simulink model "SignalProcessing3"  (R2019b)
settings: Solver=VariableStepAuto  StartTime=0.0  StopTime=5  RelTol=1e-3
libraries: dspsigops x4, dspstat3 x4, simulink x2, dspfdesign x1
settings Model: Creator=Ege  LastModifiedBy=90534
settings DataIOCC: ReturnWorkspaceOutputs=off
settings DebuggingCC: ArithmeticOperatorsInVariantConditions=warning
settings SFSimCC: SimUseLocalCustomCode=off  CustomCodeUndefinedFunction=UseInterfaceOnly
settings RTWCC: RTWUseLocalCustomCode=off
settings CodeAppCC: StateflowObjectComments=on

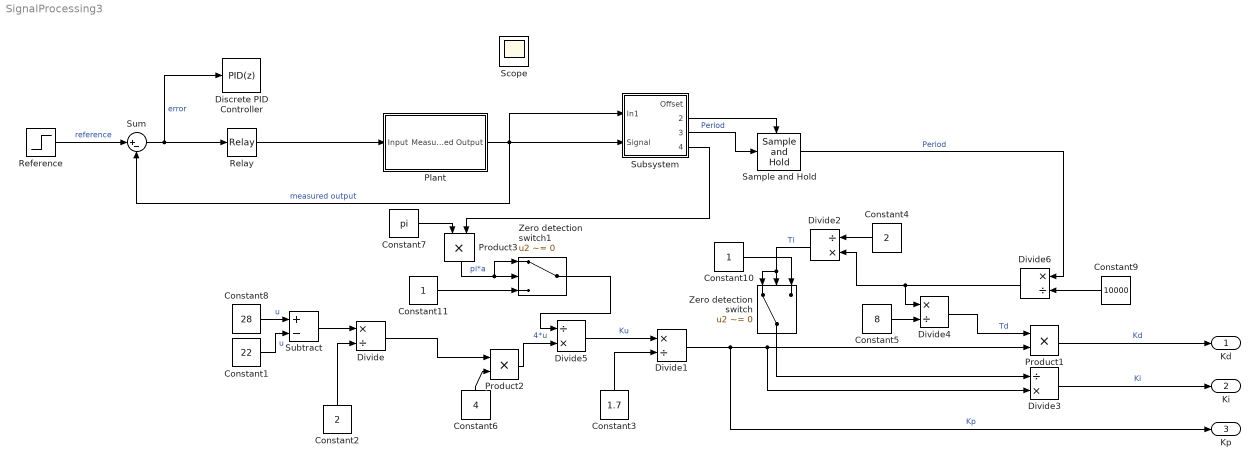
== system SignalProcessing3 ==
  Constant1 : Constant  Value=22
  Constant10 : Constant
  Constant11 : Constant
  Constant2 : Constant  Value=2
  Constant3 : Constant  Value=1.7
  Constant4 : Constant  Value=2
  Constant5 : Constant  Value=8
  Constant6 : Constant  Value=4
  Constant7 : Constant  Value=pi
  Constant8 : Constant  Value=28
  Constant9 : Constant  Value=10000
  Discrete PID Controller : simulink/Continuous/PID Controller  Controller=PID  Form=Parallel  TimeDomain=Discrete-time  SampleTime=-1  IntegratorMethod=Forward Euler  FilterMethod=Forward Euler  ControllerParametersSource=internal  P=27.5252785714347  I=242.974803591307  D=0.637793516322299  UseFilter=off  N=9773.41340021372  TunerSelectOption=Transfer Function Based (PID Tuner App)  InitialConditionSource=internal  InitialConditionForIntegrator=0  InitialConditionForFilter=0  DifferentiatorICPrevScaledInput=0  ExternalReset=none  TrackingMode=off  Kt=1  LimitOutput=off  UpperSaturationLimit=inf  LowerSaturationLimit=-inf  LinearizeAsGain=off  AntiWindupMode=none  Kb=1  POutMin=[]  POutMax=[]  IOutMin=[]  IOutMax=[]  DOutMin=[]  DOutMax=[]  NOutMin=[]  NOutMax=[]  SumOutMin=[]  SumOutMax=[]  SaturationOutMin=[]  SaturationOutMax=[]  PParamMin=[]  PParamMax=[]  IParamMin=[]  IParamMax=[]  DParamMin=[]  DParamMax=[]  NParamMin=[]  NParamMax=[]  KbParamMin=[]  KbParamMax=[]  KtParamMin=[]  KtParamMax=[]  KbOutMin=[]  KbOutMax=[]  KtOutMin=[]  KtOutMax=[]  IntegratorOutMin=[]  IntegratorOutMax=[]  FilterOutMin=[]  FilterOutMax=[]  SumI1OutMin=[]  SumI1OutMax=[]  SumI2OutMin=[]  SumI2OutMax=[]  SumI3OutMin=[]  SumI3OutMax=[]  SumI4OutMin=[]  SumI4OutMax=[]  SumDOutMin=[]  SumDOutMax=[]  DifferentiatorOutMin=[]  DifferentiatorOutMax=[]  FilterDiffOutCoefMin=[]  FilterDiffOutCoefMax=[]  ReciprocalOutMin=[]  ReciprocalOutMax=[]  SumDenOutMin=[]  SumDenOutMax=[]  SumNumOutMin=[]  SumNumOutMax=[]  DivideOutMin=[]  DivideOutMax=[]  IntegratorContinuousStateAttributes=''  IntegratorStateMustResolveToSignalObject=off  IntegratorRTWStateStorageClass=Auto  FilterContinuousStateAttributes=''  FilterStateMustResolveToSignalObject=off  FilterRTWStateStorageClass=Auto  ParallelPVariant=InternalParameters  IdealPVariant=Disabled  IVariant=InternalParameters  DVariant=InternalParameters  IntegratorVariant=Discrete  SatVariant=Disabled  AWVariant=Passthrough  PCopyVariant=Disabled  TRVariant=Disabled  FdbkBlocksVariant=Forward  IdealPFdbkVariant=Disabled  SatFdbkVariant=Disabled  DerivativeFilterVariant=Differentiator  NVariant=Passthrough  NCopyVariant=Disabled_SignalSpec  FilterICVariant=InternalICsDifferentiator  IntegratorICVariant=InternalICs  ExternalResetVariant=Disabled  TRSumVariant=Passthrough  SumFdbkVariant=Disabled  SumVariant=Sum_PID
  Divide : Product  Inputs=*/
  Divide1 : Product  Inputs=*/  SaturateOnIntegerOverflow=on  RndMeth=Zero
  Divide2 : Product  Inputs=/*  SaturateOnIntegerOverflow=on  RndMeth=Zero
  Divide3 : Product  Inputs=/*  SaturateOnIntegerOverflow=on  RndMeth=Zero
  Divide4 : Product  Inputs=*/  SaturateOnIntegerOverflow=on  RndMeth=Zero
  Divide5 : Product  Inputs=/*  SaturateOnIntegerOverflow=on  RndMeth=Zero
  Divide6 : Product  Inputs=*/
  Plant : Subsystem
  Product1 : Product
  Product2 : Product
  Product3 : Product
  Reference : Step  After=25  SampleTime=0
  Relay : Relay  OnOutputValue=on  OffOutputValue=off
  Sample and Hold : dspsigops/Sample and Hold  trig=Rising edge  initCond=0  latchinput=off
  Subsystem : Subsystem
  Subtract : Sum  Inputs=+-
  Sum : Sum  Inputs=|+-
  Zero detection switch : Switch  Criteria=u2 ~= 0
  Zero detection switch1 : Switch  Criteria=u2 ~= 0
  Kd : Outport
  "Ki " : Outport  Port=2
  Kp : Outport  Port=3
  Scope : Scope
  wires:
  Subtract/1 -> Divide/1
  Constant1/1 -> Subtract/2  "u"
  Constant8/1 -> Subtract/1  "u"
  Constant2/1 -> Divide/2
  Relay/1 -> Plant/1(Input)
  Sum/1 -> Relay/1, Discrete PID Controller/1  "error"
  Plant/1(Measured Output) -> Subsystem/2("Signal "), Subsystem/1(In1), Sum/2  "measured output"
  Reference/1 -> Sum/1  "reference"
  Constant9/1 -> Divide6/2
  Divide6/1 -> Divide2/2, Divide4/1
  Subsystem/3("Period ") -> Sample and Hold/1  "Period"
  Divide4/1 -> Product1/1  "Td"
  Constant7/1 -> Product3/1
  Product2/1 -> Divide5/2  "4*u"
  Divide2/1 -> Zero detection switch/1, Zero detection switch/2  "Ti"
  Constant4/1 -> Divide2/1
  Constant5/1 -> Divide4/2
  Divide5/1 -> Divide1/1  "Ku"
  Product1/1 -> Kd/1  "Kd"
  Divide1/1 -> Kp/1, Divide3/2, Product1/2  "Kp"
  Product3/1 -> Zero detection switch1/1, Zero detection switch1/2  "pi*a"
  Constant6/1 -> Product2/2
  Divide/1 -> Product2/1
  Constant3/1 -> Divide1/2
  Divide3/1 -> "Ki "/1  "Ki"
  Subsystem/2(Stable) -> Sample and Hold/Trigger
  Sample and Hold/1 -> Divide6/1  "Period"
  Subsystem/4(Amplitude) -> Product3/2
  Constant10/1 -> Zero detection switch/3
  Zero detection switch/1 -> Divide3/1
  Constant11/1 -> Zero detection switch1/3
  Zero detection switch1/1 -> Divide5/1

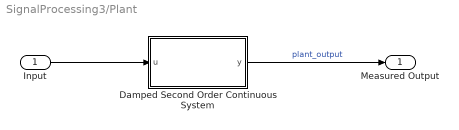
== system SignalProcessing3/Plant ==
  Input : Inport
  Damped Second Order Continuous System : Subsystem  mask{wn=90, zeta=5}
      mask prompts: wn "Undamped natural frequency (wn, rad/s)"; zeta "Damping factor (zeta)"
  Measured Output : Outport
  wires:
  Input/1 -> Damped Second Order Continuous System/1(u)
  Damped Second Order Continuous System/1(y) -> Measured Output/1  "plant_output"

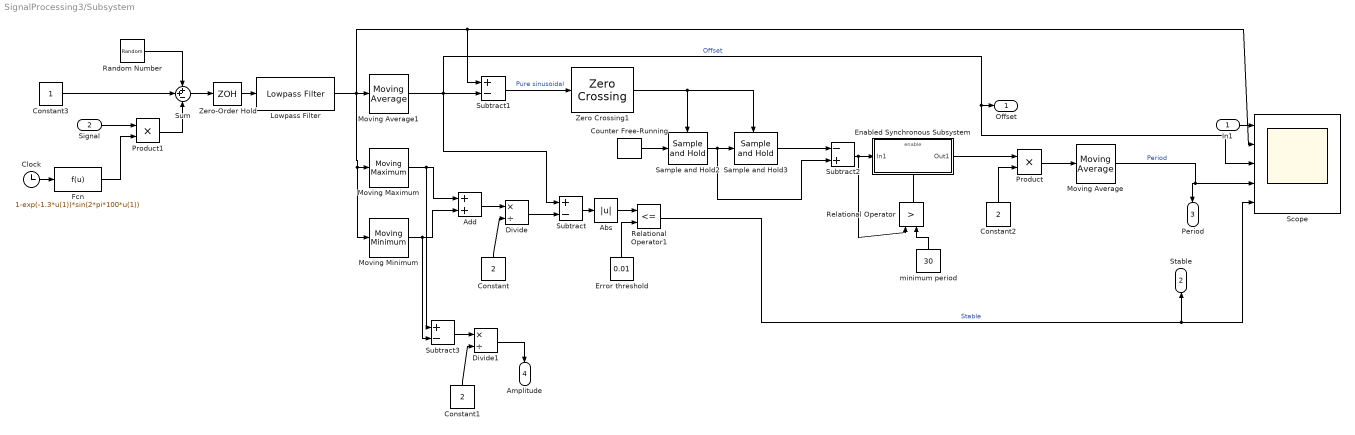
== system SignalProcessing3/Subsystem ==
  In1 : Inport
  "Signal " : Inport  Port=2
  Abs : Abs
  Add : Sum
  Clock : Clock
  Constant : Constant  Value=2
  Constant1 : Constant  Value=2
  Constant2 : Constant  Value=2
  Constant3 : Constant
  Counter Free-Running : simulink/Sources/Counter Free-Running  NumBits=16  tsamp=-1
  Divide : Product  Inputs=*/
  Divide1 : Product  Inputs=*/
  Enabled Synchronous Subsystem : Subsystem  TreatAsAtomicUnit=on
  Error threshold : Constant  Value=0.01
  Fcn : Fcn  Expr=1-exp(-1.3*u(1))*sin(2*pi*100*u(1))
  Lowpass Filter : dspfdesign/Lowpass Filter  FilterType=FIR  DesignForMinimumOrder=on  FilterOrder=50  PassbandFrequency=1e3  StopbandFrequency=2e3  PassbandRipple=0.1  StopbandAttenuation=80  InheritSampleRate=on  SampleRate=44100  SimulateUsing=Interpreted execution  roundingMode=Floor  coeffsDataTypeStr=fixdt(1,16)
  Moving Average : dspstat3/Moving Average  Method=Sliding window  ForgettingFactorPort=off  SpecifyWindowLength=on  WindowLength=10000  ForgettingFactor=0.1  SimulateUsing=Code generation
  Moving Average1 : dspstat3/Moving Average  Method=Sliding window  ForgettingFactorPort=off  SpecifyWindowLength=on  WindowLength=10000  ForgettingFactor=0.1  SimulateUsing=Code generation
  Moving Maximum : dspstat3/Moving Maximum  SpecifyWindowLength=on  WindowLength=10000  SimulateUsing=Code generation
      settings: SourceProductName=DSP System Toolbox  SourceProductBaseCode=DS
  Moving Minimum : dspstat3/Moving Minimum  SpecifyWindowLength=on  WindowLength=10000  SimulateUsing=Code generation
      settings: SourceProductName=DSP System Toolbox  SourceProductBaseCode=DS
  Product : Product
  Product1 : Product
  Random Number : RandomNumber  Variance=0.01  SampleTime=0.0001
  Relational Operator : RelationalOperator  Operator=>  OutDataTypeStr=boolean  RndMeth=Nearest
  Relational Operator1 : RelationalOperator  Operator=<=  OutDataTypeStr=boolean  RndMeth=Simplest
  Sample and Hold2 : dspsigops/Sample and Hold  trig=Rising edge  initCond=0  latchinput=on
  Sample and Hold3 : dspsigops/Sample and Hold  trig=Rising edge  initCond=0  latchinput=on
  Scope : Scope  NumInputPorts=5
  Subtract : Sum  Inputs=+-
  Subtract1 : Sum  Inputs=+-
  Subtract2 : Sum  Inputs=-+  AccumDataTypeStr=fixdt(0,16,0)
  Subtract3 : Sum  Inputs=+-
  Sum : Sum  Inputs=++-
  Zero Crossing1 : dspsigops/Zero Crossing  InputProcessing=Columns as channels (frame based)
      settings: SourceProductName=DSP System Toolbox  SourceProductBaseCode=DS
  Zero-Order Hold : ZeroOrderHold  SampleTime=0.0001
  minimum period : Constant  Value=30
  Offset : Outport
  Stable : Outport  Port=2
  "Period " : Outport  Port=3
  Amplitude : Outport  Port=4
  wires:
  Moving Maximum/1 -> Subtract3/1, Add/1
  Lowpass Filter/1 -> Moving Minimum/1, Moving Maximum/1, Moving Average1/1, Scope/2, Subtract1/1
  Moving Average1/1 -> Offset/1, Scope/3, Subtract/1, Subtract1/2  "Offset"
  Counter Free-Running/1 -> Sample and Hold2/1
  Clock/1 -> Fcn/1
  Sample and Hold2/1 -> Subtract2/2, Sample and Hold3/1
  Divide/1 -> Subtract/2
  Relational Operator1/1 -> Stable/1, Scope/5  "Stable"
  Sample and Hold3/1 -> Subtract2/1
  Subtract/1 -> Abs/1
  Constant/1 -> Divide/2
  Sum/1 -> Zero-Order Hold/1
  Product/1 -> Moving Average/1
  Enabled Synchronous Subsystem/1(Out1) -> Product/1
  Abs/1 -> Relational Operator1/1
  Zero Crossing1/1 -> Sample and Hold3/Trigger, Sample and Hold2/Trigger
  Subtract2/1 -> Enabled Synchronous Subsystem/1(In1), Relational Operator/1
  Add/1 -> Divide/1
  Random Number/1 -> Sum/1
  Fcn/1 -> Product1/2
  Constant2/1 -> Product/2
  Relational Operator/1 -> Enabled Synchronous Subsystem/Enable
  Moving Minimum/1 -> Subtract3/2, Add/2
  Error threshold/1 -> Relational Operator1/2
  minimum period/1 -> Relational Operator/2
  Subtract1/1 -> Zero Crossing1/1  "Pure sinusoidal"
  "Signal "/1 -> Product1/1
  Moving Average/1 -> "Period "/1, Scope/4  "Period"
  Zero-Order Hold/1 -> Lowpass Filter/1
  Product1/1 -> Sum/3
  Constant3/1 -> Sum/2
  In1/1 -> Scope/1
  Constant1/1 -> Divide1/2
  Subtract3/1 -> Divide1/1
  Divide1/1 -> Amplitude/1

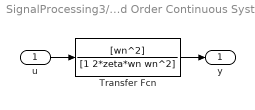
== system SignalProcessing3/Plant/Damped Second Order Continuous System ==
  u : Inport
  Transfer Fcn : TransferFcn  Numerator=[wn^2]  Denominator=[1 2*zeta*wn wn^2]
  y : Outport
  wires:
  Transfer Fcn/1 -> y/1
  u/1 -> Transfer Fcn/1

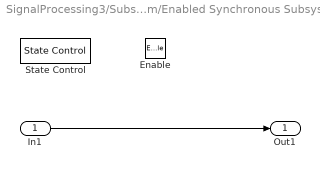
== system SignalProcessing3/Subsystem/Enabled Synchronous Subsystem ==
  In1 : Inport
  Enable : EnablePort
  State Control : StateControl
  Out1 : Outport
  wires:
  In1/1 -> Out1/1
